simulink model "Controller"  (R2021a)
settings: Solver=VariableStepAuto  StartTime=0.0  StopTime=10.0  RelTol=1e-3
settings Model: Creator=osama  LastModifiedBy=yehia
settings SolverCC: AlgebraicLoopSolver=TrustRegion
settings DataIOCC: ReturnWorkspaceOutputs=off
settings DebuggingCC: SFMachineParentedDataDiag=warning  ArithmeticOperatorsInVariantConditions=warning
settings SFSimCC: SimUseLocalCustomCode=off  CustomCodeUndefinedFunction=UseInterfaceOnly
settings RTWCC: RTWUseLocalCustomCode=off
settings CodeAppCC: StateflowObjectComments=on

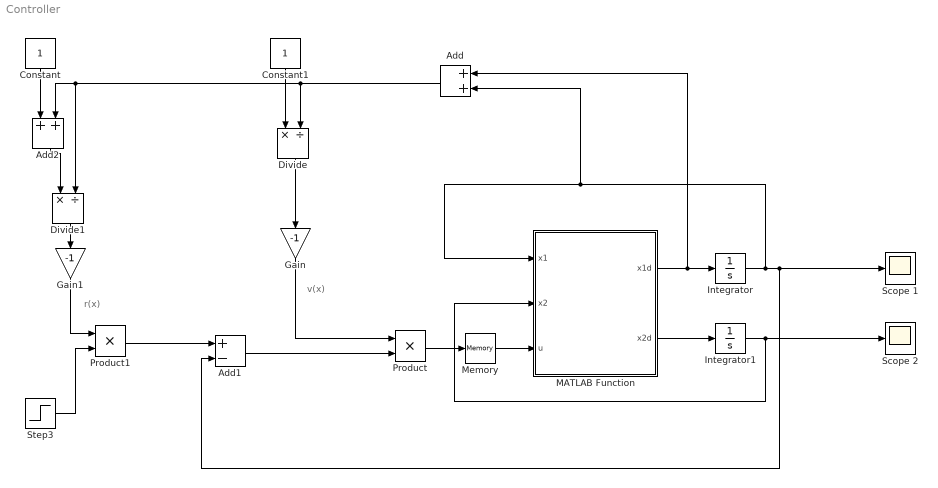
== system Controller ==
  note: r(x)
  note: v(x)
  Add : Sum
  Add1 : Sum  Inputs=+-
  Add2 : Sum
  Constant : Constant
  Constant1 : Constant
  Divide : Product  Inputs=*/
  Divide1 : Product  Inputs=*/
  Gain : Gain  Gain=-1
  Gain1 : Gain  Gain=-1
  Integrator : Integrator  InitialCondition=1
  Integrator1 : Integrator  InitialCondition=1
  MATLAB Function : MATLAB Function  TreatAsAtomicUnit=on
  Memory : Memory  InitialCondition=1  LinearizeMemory=on
  Product : Product
  Product1 : Product
  Scope 1 : Scope
  Scope 2 : Scope
  Step3 : Step  SampleTime=0
  wires:
  MATLAB Function/1(x1d) -> Add/1, Integrator/1
  MATLAB Function/2(x2d) -> Integrator1/1
  Integrator/1 -> Add1/2, Scope 1/1, Add/2, MATLAB Function/1(x1)
  Integrator1/1 -> Scope 2/1, MATLAB Function/2(x2)
  Add/1 -> Divide/2, Add2/2, Divide1/2
  Constant1/1 -> Divide/1
  Product/1 -> Memory/1
  Add1/1 -> Product/2
  Divide/1 -> Gain/1
  Gain/1 -> Product/1
  Add2/1 -> Divide1/1
  Constant/1 -> Add2/1
  Divide1/1 -> Gain1/1
  Gain1/1 -> Product1/1
  Step3/1 -> Product1/2
  Product1/1 -> Add1/1
  Memory/1 -> MATLAB Function/3(u)

== matlab function Controller/MATLAB Function ==
  data: x1 input; x2 input; x1d output; x2d output; u input
function [x1d,x2d]=fcn(x1,x2,u)
x1d=(2*x2*x1)/(.06+x2+.3*x2^(2))-x1*u;
x2d=((-1/.7)*(2*x2*x1))/(.06+x2+.3*x2^(2))-(2-x2)*u;
